simulink model "Subsystem10"  (R2020b)
settings: Solver=VariableStepAuto  StartTime=0.0  StopTime=10.0  RelTol=1e-3
model workspace (MAT data in the model file):
  a = Simulink.Parameter
  a.Value = 1
  a.DataType = 'auto'
  a.Dimensions = [1 1]
  b = Simulink.Parameter
  b.Value = 2
  b.DataType = 'auto'
  b.Dimensions = [1 1]
  c = Simulink.Parameter
  c.Value = -3
  c.DataType = 'auto'
  c.Dimensions = [1 1]
  d = Simulink.Parameter
  d.Value = -4
  d.DataType = 'auto'
  d.Dimensions = [1 1]
  e = Simulink.Parameter
  e.Value = 5
  e.DataType = 'auto'
  e.Dimensions = [1 1]
settings Model: Creator=sushma  LastModifiedBy=sushma
settings DataIOCC: SaveOutput=off  SaveTime=off

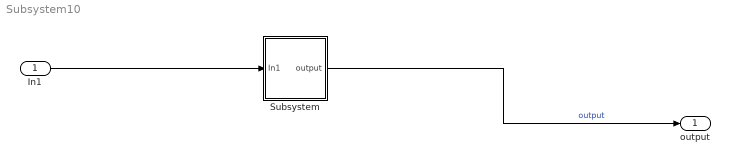
== system Subsystem10 ==
  In1 : Inport  OutDataTypeStr=double  PortDimensions=1  SampleTime=0
  Subsystem : Subsystem
  output : Outport  OutDataTypeStr=double  PortDimensions=1  SampleTime=0
  wires:
  Subsystem/1(output) -> output/1  "output"
  In1/1 -> Subsystem/1(In1)

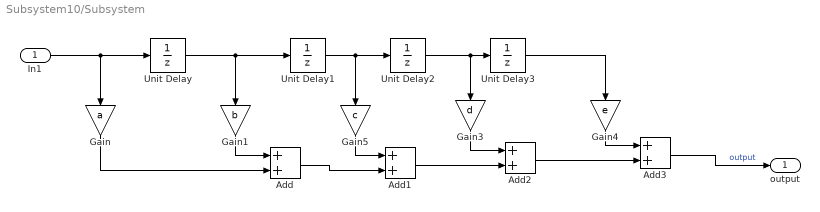
== system Subsystem10/Subsystem ==
  In1 : Inport
  Add{,1..3} (4 alike) : Sum
  Gain : Gain  Gain=a
  Gain1 : Gain  Gain=b
  Gain3 : Gain  Gain=d
  Gain4 : Gain  Gain=e
  Gain5 : Gain  Gain=c
  Unit Delay{,1..3} (4 alike) : UnitDelay  SampleTime=-1  HasFrameUpgradeWarning=on
  output : Outport
  wires:
  Add/1 -> Add1/2
  Gain5/1 -> Add1/1
  Unit Delay/1 -> Unit Delay1/1, Gain1/1
  Unit Delay3/1 -> Gain4/1
  Gain1/1 -> Add/1
  Gain4/1 -> Add3/1
  Unit Delay2/1 -> Unit Delay3/1, Gain3/1
  Gain/1 -> Add/2
  Add1/1 -> Add2/2
  Unit Delay1/1 -> Unit Delay2/1, Gain5/1
  In1/1 -> Gain/1, Unit Delay/1
  Gain3/1 -> Add2/1
  Add2/1 -> Add3/2
  Add3/1 -> output/1  "output"
